simulink model "Pthmodel"  (R2020a)
settings: Solver=VariableStepAuto  StartTime=0.0  StopTime=10.0  RelTol=1e-3
values from neighbouring files (symbols this model uses):
  beta = 0.0067    [simplified_reactor_core_main.m]
  mean_prompt_neutron_gen_t = 0.07669    [simplified_reactor_core_main.m]
settings Model: Creator=marce  LastModifiedBy=tkdmc

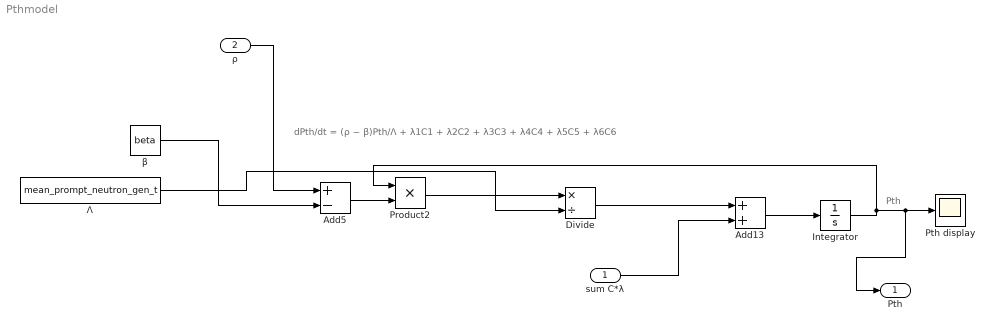
== system Pthmodel ==
  note: Pth
  note: dPth/dt = (ρ − β)Pth/Λ + λ1C1 + λ2C2 + λ3C3 + λ4C4 + λ5C5 + λ6C6
  sum C*λ : Inport
  ρ : Inport  Port=2
  Add13 : Sum
  Add5 : Sum  Inputs=+-
  Divide : Product  Inputs=*/
  Integrator : Integrator  InitialCondition=1
  Product2 : Product
  Pth display : Scope
  "Λ " : Constant  Value=mean_prompt_neutron_gen_t
  β : Constant  Value=beta
  Pth : Outport
  wires:
  "Λ "/1 -> Divide/2
  Product2/1 -> Divide/1
  Divide/1 -> Add13/1
  β/1 -> Add5/2
  Add13/1 -> Integrator/1
  Add5/1 -> Product2/2
  Integrator/1 -> Pth/1, Pth display/1, Product2/1
  sum C*λ/1 -> Add13/2
  ρ/1 -> Add5/1
